simulink model "tb_CameraIO"  (R2022b)
settings: Solver=FixedStepDiscrete  StartTime=0  StopTime=0.0001  RelTol=1e-3
InitFcn:
  | init_CameraIO;
values from neighbouring files (symbols this model uses):
  AXI_CameraIO_Control = Simulink.Parameter    [init_CameraIO.m]
  model_time_step = 1/80e6    (= 1.25e-08)    [init_CameraIO.m]    (also in init_SYSTEM.m)
libraries: simulink x45, hdlsllib x13
Description:
  | Copyright (c) 2023, Alexei Evsenin, evsenin@gmail.com
settings Model: DataTypeOverride=Off  PacingRate=0.011000  Creator=mmwoperator  LastModifiedBy=evsenin
settings SolverCC: AlgebraicLoopSolver=TrustRegion
settings DataIOCC: SaveOutput=off  DSMLogging=off  SaveTime=off  ReturnWorkspaceOutputs=off
settings OptimizationCC: BlockReduction=off  ConditionallyExecuteInputs=off  DefaultParameterBehavior=Inlined  InheritOutputTypeSmallerThanSingle=on  DefaultUnderspecifiedDataType=single
settings DebuggingCC: AlgebraicLoopMsg=error  SingleTaskRateTransMsg=error  ParameterUnderflowMsg=error  ParameterPrecisionLossMsg=none  ParameterTunabilityLossMsg=error  FixptConstUnderflowMsg=warning  FixptConstOverflowMsg=warning  UnconnectedInputMsg=warning  UnconnectedOutputMsg=warning  UnconnectedLineMsg=warning  SFMachineParentedDataDiag=warning  UnderSpecifiedDimensionMsg=warning
settings HardwareCC: ProdBitPerPointer=32  ProdBitPerSizeT=32  ProdBitPerPtrDiffT=32  ProdLargestAtomicFloat=None  ProdIntDivRoundTo=Undefined  ProdEndianess=Unspecified  ProdWordSize=32  ProdHWDeviceType=ASIC/FPGA->ASIC/FPGA  TargetBitPerPointer=64  TargetBitPerSizeT=64  TargetBitPerPtrDiffT=64  TargetLongLongMode=on  TargetIntDivRoundTo=Zero  TargetEndianess=LittleEndian  TargetWordSize=64  TargetHWDeviceType=Custom Processor->MATLAB Host Computer  ProdEqTarget=off
settings ModelReferenceCC: EnableRefExpFcnMdlSchedulingChecks=on
settings RTWCC: DLArmComputeVersion=19.05

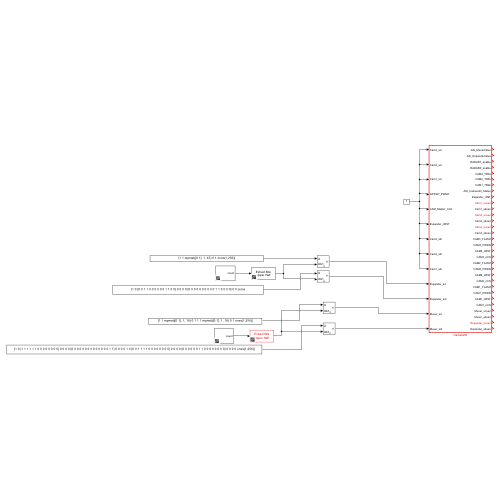
[thumbnail: Simulink's stored preview of the top-level diagram]
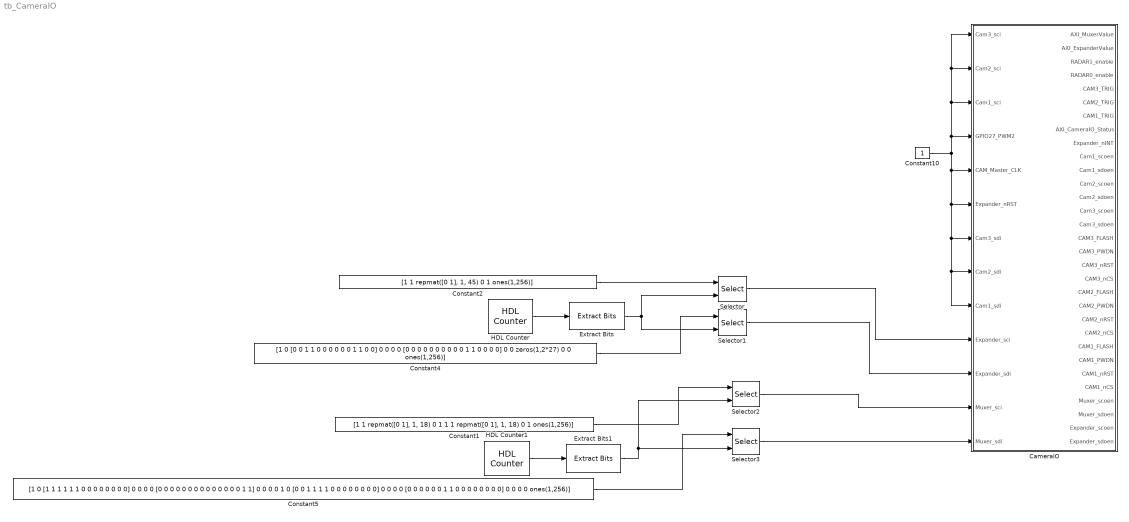
== system tb_CameraIO ==
  CameraIO : Subsystem  TreatAsAtomicUnit=on  SystemSampleTime=model_time_step
      settings: RTWSystemCode=Inline
  Constant1 : Constant  Value=[1 1 repmat([0 1], 1, 18) 0 1 1 1 repmat([0 1], 1, 18) 0 1 ones(1,256)]  OutDataTypeStr=boolean  SampleTime=model_time_step
  Constant10 : Constant  OutDataTypeStr=boolean  SampleTime=-1
  Constant2 : Constant  Value=[1 1 repmat([0 1], 1, 45) 0 1 ones(1,256)]  OutDataTypeStr=boolean  SampleTime=model_time_step
  Constant4 : Constant  Value="[1 0 [0 0 1 1 0 0 0 0 0 0 1 1 0 0] 0 0 0 0 [0 0 0 0 0 0 0 0 0 0 1 1 0 0 0 0] 0 0 zeros(1,2*27)  0 0 ones(1,256)]"  OutDataTypeStr=boolean  SampleTime=model_time_step
  Constant5 : Constant  Value=[1 0 [1 1 1 1 1 1 0 0 0 0 0 0 0 0] 0 0 0 0 [0 0 0 0 0 0 0 0 0 0 0 0 0 0 1 1] 0 0 0 0 1 0 [0 0 1 1 1 1 0 0 0 0 0 0 0 0] 0 0 0 0 [0 0 0 0 0 0 1 1 0 0 0 0 0 0 0 0] 0 0 0 0 ones(1,256)]  OutDataTypeStr=boolean  SampleTime=model_time_step
  Extract Bits : simulink/Logic and Bit Operations/Extract Bits  bitsToExtract=Upper half  numBits=8  bitIdxRange=[0 7]  outScalingMode=Treat bit field as an integer
  Extract Bits1 : simulink/Logic and Bit Operations/Extract Bits  bitsToExtract=Upper half  numBits=8  bitIdxRange=[0 7]  outScalingMode=Treat bit field as an integer
  HDL Counter : hdlsllib/Sources/HDL Counter  CountType=Free running  CountInit=0  CountStep=1  CountMax=25  CountFromType=Initial value  CountFrom=0  CountResetPort=off  CountLoadPort=off  CountEnbPort=off  CountDirPort=off  CountHitOutputPort=off  CountDataType=Unsigned  CountWordLen=16  CountFracLen=0  CountSampTime=model_time_step
  HDL Counter1 : hdlsllib/Sources/HDL Counter  CountType=Free running  CountInit=0  CountStep=1  CountMax=25  CountFromType=Initial value  CountFrom=0  CountResetPort=off  CountLoadPort=off  CountEnbPort=off  CountDirPort=off  CountHitOutputPort=off  CountDataType=Unsigned  CountWordLen=16  CountFracLen=0  CountSampTime=model_time_step
  Selector{,1..3} (4 alike) : Selector  IndexMode=Zero-based  IndexOptions=Index vector (port)  Indices=[1 3]  OutputSizes=1
  wires:
  Constant2/1 -> Selector/1
  Selector/1 -> CameraIO/4(Expander_sci)
  Selector1/1 -> CameraIO/3(Expander_sdi)
  Extract Bits/1 -> Selector1/2, Selector/2
  Constant4/1 -> Selector1/1
  HDL Counter/1 -> Extract Bits/1
  Extract Bits1/1 -> Selector3/2, Selector2/2
  Selector3/1 -> CameraIO/1(Muxer_sdi)
  Selector2/1 -> CameraIO/2(Muxer_sci)
  Constant1/1 -> Selector2/1
  Constant5/1 -> Selector3/1
  HDL Counter1/1 -> Extract Bits1/1
  Constant10/1 -> CameraIO/5(Cam1_sdi), CameraIO/6(Cam2_sdi), CameraIO/7(Cam3_sdi), CameraIO/8(Expander_nRST), CameraIO/9(CAM_Master_CLK), CameraIO/13(Cam3_sci), CameraIO/12(Cam2_sci), CameraIO/11(Cam1_sci), CameraIO/10(GPIO27_PWM2)

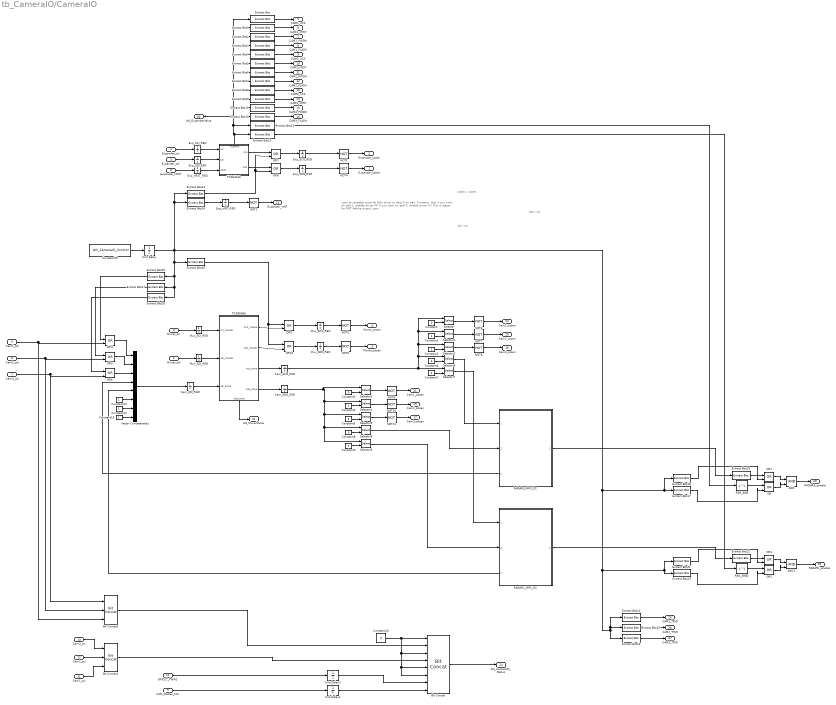
== system tb_CameraIO/CameraIO ==
  note: sdoen /
      | scoen
  note: _oen pin enables external bidir driver to pass 0 on pad.
      | It means, that
      | if you want on pad 1, disable driver (0)
      | if you want on pad 0, enable driver (1)
      | This is reason for NOT before output _oen
  note: sdi /
      | sci
  note: sda /
      | scl
  Muxer_sdi : Inport
  Muxer_sci : Inport  Port=2
  Expander_sdi : Inport  Port=3
  Expander_sci : Inport  Port=4
  Cam1_sdi : Inport  Port=5
  Cam2_sdi : Inport  Port=6
  Cam3_sdi : Inport  Port=7
  Expander_nRST : Inport  Port=8
  CAM_Master_CLK : Inport  Port=9
  GPIO27_PWM2 : Inport  Port=10
  Cam1_sci : Inport  Port=11
  Cam2_sci : Inport  Port=12
  Cam3_sci : Inport  Port=13
  AND : Logic  IconShape=distinctive  AllPortsSameDT=off  OutDataTypeStr=boolean
  AND1 : Logic  IconShape=distinctive  AllPortsSameDT=off  OutDataTypeStr=boolean
  Bit Concat : hdlsllib/Logic and Bit Operations/Bit Concat  numInputs=8
  Bit Concat1 : hdlsllib/Logic and Bit Operations/Bit Concat  numInputs=3
  Bit Concat2 : hdlsllib/Logic and Bit Operations/Bit Concat  numInputs=3
  Cam_SCO_REG : UnitDelay  SampleTime=-1  HasFrameUpgradeWarning=on
  Cam_SDI_REG : UnitDelay  SampleTime=-1  HasFrameUpgradeWarning=on
  Cam_SDO_REG : UnitDelay  SampleTime=-1  HasFrameUpgradeWarning=on
  Constant : Constant  Value=0  OutDataTypeStr=uint8  SampleTime=-1
  Constant1 : Constant  OutDataTypeStr=uint8  SampleTime=-1
  Constant10 : Constant  Value=0  OutDataTypeStr=boolean  SampleTime=-1
  Constant13 : Constant  OutDataTypeStr=boolean  SampleTime=-1
  Constant14 : Constant  OutDataTypeStr=boolean  SampleTime=-1
  Constant15 : Constant  OutDataTypeStr=boolean  SampleTime=-1
  Constant19 : Constant  Value=AXI_CameraIO_Control  SampleTime=-1
  Constant2 : Constant  Value=2  OutDataTypeStr=uint8  SampleTime=-1
  Constant3 : Constant  Value=0  OutDataTypeStr=uint8  SampleTime=-1
  Constant4 : Constant  OutDataTypeStr=uint8  SampleTime=-1
  Constant5 : Constant  Value=2  OutDataTypeStr=uint8  SampleTime=-1
  Constant6 : Constant  Value=3  OutDataTypeStr=uint8  SampleTime=-1
  Constant7 : Constant  Value=4  OutDataTypeStr=uint8  SampleTime=-1
  Constant8 : Constant  Value=3  OutDataTypeStr=uint8  SampleTime=-1
  Constant9 : Constant  Value=4  OutDataTypeStr=uint8  SampleTime=-1
  Exp_SCI_REG : UnitDelay  SampleTime=-1  HasFrameUpgradeWarning=on
  Exp_SCO_REG : UnitDelay  SampleTime=-1  HasFrameUpgradeWarning=on
  Exp_SDI_REG : UnitDelay  SampleTime=-1  HasFrameUpgradeWarning=on
  Exp_SDO_REG : UnitDelay  SampleTime=-1  HasFrameUpgradeWarning=on
  Exp_nINT_REG : UnitDelay  SampleTime=-1  HasFrameUpgradeWarning=on
  Exp_nRST_REG : UnitDelay  SampleTime=-1  HasFrameUpgradeWarning=on
  Extract Bits : simulink/Logic and Bit Operations/Extract Bits  bitsToExtract=Range of bits  numBits=8  bitIdxRange=0  outScalingMode=Treat bit field as an integer
  Extract Bits1 : simulink/Logic and Bit Operations/Extract Bits  bitsToExtract=Range of bits  numBits=8  bitIdxRange=1  outScalingMode=Treat bit field as an integer
  Extract Bits10 : simulink/Logic and Bit Operations/Extract Bits  bitsToExtract=Range of bits  numBits=8  bitIdxRange=11  outScalingMode=Treat bit field as an integer
  Extract Bits11 : simulink/Logic and Bit Operations/Extract Bits  bitsToExtract=Range of bits  numBits=8  bitIdxRange=12  outScalingMode=Treat bit field as an integer
  Extract Bits12 : simulink/Logic and Bit Operations/Extract Bits  bitsToExtract=Range of bits  numBits=8  bitIdxRange=13  outScalingMode=Treat bit field as an integer
  Extract Bits13 : simulink/Logic and Bit Operations/Extract Bits  bitsToExtract=Range of bits  numBits=8  bitIdxRange=14  outScalingMode=Treat bit field as an integer
  Extract Bits14 : simulink/Logic and Bit Operations/Extract Bits  bitsToExtract=Range of bits  numBits=8  bitIdxRange=1  outScalingMode=Treat bit field as an integer
  Extract Bits15 : simulink/Logic and Bit Operations/Extract Bits  bitsToExtract=Range of bits  numBits=8  bitIdxRange=2  outScalingMode=Treat bit field as an integer
  Extract Bits16 : simulink/Logic and Bit Operations/Extract Bits  bitsToExtract=Range of bits  numBits=8  bitIdxRange=3  outScalingMode=Treat bit field as an integer
  Extract Bits17 : simulink/Logic and Bit Operations/Extract Bits  bitsToExtract=Range of bits  numBits=8  bitIdxRange=10  outScalingMode=Treat bit field as an integer
  Extract Bits18 : simulink/Logic and Bit Operations/Extract Bits  bitsToExtract=Range of bits  numBits=8  bitIdxRange=11  outScalingMode=Treat bit field as an integer
  Extract Bits19 : simulink/Logic and Bit Operations/Extract Bits  bitsToExtract=Range of bits  numBits=8  bitIdxRange=0  outScalingMode=Treat bit field as an integer
  Extract Bits2 : simulink/Logic and Bit Operations/Extract Bits  bitsToExtract=Range of bits  numBits=8  bitIdxRange=2  outScalingMode=Treat bit field as an integer
  Extract Bits20 : simulink/Logic and Bit Operations/Extract Bits  bitsToExtract=Range of bits  numBits=8  bitIdxRange=8  outScalingMode=Treat bit field as an integer
  Extract Bits21 : simulink/Logic and Bit Operations/Extract Bits  bitsToExtract=Range of bits  numBits=8  bitIdxRange=9  outScalingMode=Treat bit field as an integer
  Extract Bits22 : simulink/Logic and Bit Operations/Extract Bits  bitsToExtract=Range of bits  numBits=8  bitIdxRange=0  outScalingMode=Treat bit field as an integer
  Extract Bits23 : simulink/Logic and Bit Operations/Extract Bits  bitsToExtract=Range of bits  numBits=8  bitIdxRange=16  outScalingMode=Treat bit field as an integer
  Extract Bits24 : simulink/Logic and Bit Operations/Extract Bits  bitsToExtract=Range of bits  numBits=8  bitIdxRange=17  outScalingMode=Treat bit field as an integer
  Extract Bits25 : simulink/Logic and Bit Operations/Extract Bits  bitsToExtract=Range of bits  numBits=8  bitIdxRange=24  outScalingMode=Treat bit field as an integer
  Extract Bits26 : simulink/Logic and Bit Operations/Extract Bits  bitsToExtract=Range of bits  numBits=8  bitIdxRange=20  outScalingMode=Treat bit field as an integer
  Extract Bits27 : simulink/Logic and Bit Operations/Extract Bits  bitsToExtract=Range of bits  numBits=8  bitIdxRange=25  outScalingMode=Treat bit field as an integer
  Extract Bits28 : simulink/Logic and Bit Operations/Extract Bits  bitsToExtract=Range of bits  numBits=8  bitIdxRange=26  outScalingMode=Treat bit field as an integer
  Extract Bits3 : simulink/Logic and Bit Operations/Extract Bits  bitsToExtract=Range of bits  numBits=8  bitIdxRange=3  outScalingMode=Treat bit field as an integer
  Extract Bits4 : simulink/Logic and Bit Operations/Extract Bits  bitsToExtract=Range of bits  numBits=8  bitIdxRange=5  outScalingMode=Treat bit field as an integer
  Extract Bits5 : simulink/Logic and Bit Operations/Extract Bits  bitsToExtract=Range of bits  numBits=8  bitIdxRange=6  outScalingMode=Treat bit field as an integer
  Extract Bits6 : simulink/Logic and Bit Operations/Extract Bits  bitsToExtract=Range of bits  numBits=8  bitIdxRange=7  outScalingMode=Treat bit field as an integer
  Extract Bits7 : simulink/Logic and Bit Operations/Extract Bits  bitsToExtract=Range of bits  numBits=8  bitIdxRange=8  outScalingMode=Treat bit field as an integer
  Extract Bits8 : simulink/Logic and Bit Operations/Extract Bits  bitsToExtract=Range of bits  numBits=8  bitIdxRange=9  outScalingMode=Treat bit field as an integer
  Extract Bits9 : simulink/Logic and Bit Operations/Extract Bits  bitsToExtract=Range of bits  numBits=8  bitIdxRange=10  outScalingMode=Treat bit field as an integer
  Mux_SCI_REG : UnitDelay  SampleTime=-1  HasFrameUpgradeWarning=on
  Mux_SCO_REG : UnitDelay  SampleTime=-1  HasFrameUpgradeWarning=on
  Mux_SDI_REG : UnitDelay  SampleTime=-1  HasFrameUpgradeWarning=on
  Mux_SDO_REG : UnitDelay  SampleTime=-1  HasFrameUpgradeWarning=on
  NOT{1..11} (11 alike) : Logic  Operator=NOT  IconShape=distinctive  AllPortsSameDT=off  OutDataTypeStr=boolean
  OR{,1..10} (11 alike) : Logic  Operator=OR  IconShape=distinctive  AllPortsSameDT=off  OutDataTypeStr=boolean
  RADAR0_MIPI_I2C : Subsystem  ReferencedSubsystem=RADAR_MIPI_I2C
      settings: PortSchema="{\"entries\":[{\"content\":{\"sides\":[{\"content\":{\"connectorIds\":[\"In1\",\"In2\",\"Out2\"]},\"type\":\"ConnectorPlacement.EquallySpacedRectSide\",\"uuid\":\"b2debd9d-8b2d-4c2a-b7ea-d85f4bcb52c2\"},{\"content\":{\"connectorIds\":[\"Out1\"],\"side\":\"RIGHT\"},\"type\":\"ConnectorPlacement.EquallySpacedRectSide\",\"uuid\":\"751dea3d-0503-49a0-b2b7-e7f0bb60b899\"},{\"content\":{\"connectorIds\":[],\"side\":\"TOP\"},\"type\":\"ConnectorPlacement.EquallySpacedRectSide\",\"uuid\":\"f461e2eb-1348-46d1-881b-f4de32057164\"}]},\"type\":\"ConnectorPlacement.EquallySpacedConnector\",\"uuid\":\"9a0ee4b4-c8e7-4064-9f6e-581825dbb5da\"}],\"packageUris\":[\"http://schema.mathworks.com/mf0/Connector/R2020b\"],\"version\":\"1.0\"}"
  RADAR1_MIPI_I2C : Subsystem  ReferencedSubsystem=RADAR_MIPI_I2C
      settings: PortSchema="{\"entries\":[{\"content\":{\"sides\":[{\"content\":{\"connectorIds\":[\"In1\",\"In2\",\"Out2\"]},\"type\":\"ConnectorPlacement.EquallySpacedRectSide\",\"uuid\":\"b2debd9d-8b2d-4c2a-b7ea-d85f4bcb52c2\"},{\"content\":{\"connectorIds\":[\"Out1\"],\"side\":\"RIGHT\"},\"type\":\"ConnectorPlacement.EquallySpacedRectSide\",\"uuid\":\"751dea3d-0503-49a0-b2b7-e7f0bb60b899\"},{\"content\":{\"connectorIds\":[],\"side\":\"TOP\"},\"type\":\"ConnectorPlacement.EquallySpacedRectSide\",\"uuid\":\"f461e2eb-1348-46d1-881b-f4de32057164\"}]},\"type\":\"ConnectorPlacement.EquallySpacedConnector\",\"uuid\":\"9a0ee4b4-c8e7-4064-9f6e-581825dbb5da\"}],\"packageUris\":[\"http://schema.mathworks.com/mf0/Connector/R2020b\"],\"version\":\"1.0\"}"
  REG_ENB : Delay  DelayLength=1
  REG_ENB1 : Delay  DelayLength=1
  Selector{,1..9} (10 alike) : Selector  IndexMode=Zero-based  IndexOptions=Index vector (port)  Indices=0  OutputSizes=1
  TCA6424A : Subsystem
      settings: PortSchema="{\"entries\":[{\"content\":{\"sides\":[{\"content\":{\"connectorIds\":[\"In1\",\"In2\",\"In3\"]},\"type\":\"ConnectorPlacement.EquallySpacedRectSide\",\"uuid\":\"1d77250f-43b6-4386-b675-1e83793e08db\"},{\"content\":{\"connectorIds\":[\"Out1\",\"Out2\"],\"side\":\"RIGHT\"},\"type\":\"ConnectorPlacement.EquallySpacedRectSide\",\"uuid\":\"1b640580-4115-4d83-96ca-02609d981243\"},{\"content\":{\"connectorIds\":[\"Out3\"],\"side\":\"TOP\"},\"type\":\"ConnectorPlacement.EquallySpacedRectSide\",\"uuid\":\"6f49e433-be00-44ee-960e-7edaa7f3e149\"},{\"content\":{\"connectorIds\":[],\"side\":\"BOTTOM\"},\"type\":\"ConnectorPlacement.EquallySpacedRectSide\",\"uuid\":\"6a3152cf-8f3f-4f35-b098-7ea6aba78185\"}]},\"type\":\"ConnectorPlacement.EquallySpacedConnector\",\"uuid\":\"cd4e3591-6f3d-41af-8f32-177195735550\"}],\"packageUris\":[\"http://schema.mathworks.com/mf0/Connector/R2020b\"],\"version\":\"1.0\"}"
  TCA9548A : Subsystem
      settings: PortSchema="{\"entries\":[{\"content\":{\"sides\":[{\"content\":{\"connectorIds\":[\"In1\",\"In2\",\"In3\"]},\"type\":\"ConnectorPlacement.EquallySpacedRectSide\",\"uuid\":\"30138089-1687-4fa9-aa54-8d9fb6e280a7\"},{\"content\":{\"connectorIds\":[\"Out1\",\"Out2\",\"Out3\",\"Out4\"],\"side\":\"RIGHT\"},\"type\":\"ConnectorPlacement.EquallySpacedRectSide\",\"uuid\":\"5e979874-09c9-45f9-a69c-4ffe93cd782d\"},{\"content\":{\"connectorIds\":[],\"side\":\"TOP\"},\"type\":\"ConnectorPlacement.EquallySpacedRectSide\",\"uuid\":\"c2d29317-3627-4549-aad4-654ad2aeb24a\"},{\"content\":{\"connectorIds\":[\"Out5\"],\"side\":\"BOTTOM\"},\"type\":\"ConnectorPlacement.EquallySpacedRectSide\",\"uuid\":\"d73dba4d-9b9b-4bcf-9d79-4dc188f6521f\"}]},\"type\":\"ConnectorPlacement.EquallySpacedConnector\",\"uuid\":\"ba77235e-1c79-4f82-b9b9-043309a3d168\"}],\"packageUris\":[\"http://schema.mathworks.com/mf0/Connector/R2020b\"],\"version\":\"1.0\"}"
  Unit Delay : UnitDelay  SampleTime=-1  HasFrameUpgradeWarning=on
  Unit Delay1 : UnitDelay  SampleTime=-1  HasFrameUpgradeWarning=on
  Unit Delay2 : UnitDelay  SampleTime=-1  HasFrameUpgradeWarning=on
  Vector Concatenate1 : Concatenate  NumInputs=8
  Expander_sdoen : Outport
  Expander_scoen : Outport  Port=2
  Muxer_sdoen : Outport  Port=3
  Muxer_scoen : Outport  Port=4
  CAM1_nCS : Outport  Port=5
  CAM1_nRST : Outport  Port=6
  CAM1_PWDN : Outport  Port=7
  CAM1_FLASH : Outport  Port=8
  CAM2_nCS : Outport  Port=9
  CAM2_nRST : Outport  Port=10
  CAM2_PWDN : Outport  Port=11
  CAM2_FLASH : Outport  Port=12
  CAM3_nCS : Outport  Port=13
  CAM3_nRST : Outport  Port=14
  CAM3_PWDN : Outport  Port=15
  CAM3_FLASH : Outport  Port=16
  Cam3_sdoen : Outport  Port=17
  Cam3_scoen : Outport  Port=18
  Cam2_sdoen : Outport  Port=19
  Cam2_scoen : Outport  Port=20
  Cam1_sdoen : Outport  Port=21
  Cam1_scoen : Outport  Port=22
  Expander_nINT : Outport  Port=23
  AXI_CameraIO_Status : Outport  Port=24
  CAM1_TRIG : Outport  Port=25
  CAM2_TRIG : Outport  Port=26
  CAM3_TRIG : Outport  Port=27
  RADAR0_enable : Outport  Port=28
  RADAR1_enable : Outport  Port=29
  AXI_ExpanderValue : Outport  Port=30
  AXI_MuxerValue : Outport  Port=31
  wires:
  Expander_sci/1 -> Exp_SCI_REG/1
  Expander_sdi/1 -> Exp_SDI_REG/1
  Muxer_sci/1 -> Mux_SCI_REG/1
  Muxer_sdi/1 -> Mux_SDI_REG/1
  Extract Bits/1 -> CAM1_nCS/1
  Extract Bits1/1 -> CAM1_nRST/1
  Extract Bits2/1 -> CAM1_PWDN/1
  Extract Bits3/1 -> CAM1_FLASH/1
  Extract Bits6/1 -> CAM2_PWDN/1
  Extract Bits7/1 -> CAM2_FLASH/1
  Extract Bits5/1 -> CAM2_nRST/1
  Extract Bits4/1 -> CAM2_nCS/1
  Extract Bits9/1 -> CAM3_nRST/1
  Extract Bits10/1 -> CAM3_PWDN/1
  Extract Bits8/1 -> CAM3_nCS/1
  Extract Bits11/1 -> CAM3_FLASH/1
  Extract Bits13/1 -> REG_ENB1/1
  Extract Bits12/1 -> REG_ENB/1
  TCA6424A/3(OutPort) -> AXI_ExpanderValue/1, Extract Bits/1, Extract Bits1/1, Extract Bits2/1, Extract Bits3/1, Extract Bits4/1, Extract Bits5/1, Extract Bits6/1, Extract Bits7/1, Extract Bits8/1, Extract Bits9/1, Extract Bits10/1, Extract Bits11/1, Extract Bits12/1, Extract Bits13/1
  Selector/1 -> NOT6/1
  Constant/1 -> Selector/2
  Constant1/1 -> Selector1/2
  Selector1/1 -> NOT7/1
  Selector2/1 -> NOT8/1
  Constant2/1 -> Selector2/2
  Constant5/1 -> Selector5/2
  Constant3/1 -> Selector3/2
  Selector3/1 -> NOT9/1
  Constant4/1 -> Selector4/2
  Selector5/1 -> NOT11/1
  Selector4/1 -> NOT10/1
  TCA9548A/3(sco_slave) -> Cam_SCO_REG/1
  Constant7/1 -> Selector7/2
  Constant6/1 -> Selector6/2
  TCA9548A/4(sdo_slave) -> Cam_SDO_REG/1
  Constant8/1 -> Selector8/2
  Constant9/1 -> Selector9/2
  Constant13/1 -> Vector Concatenate1/6
  Cam3_sdi/1 -> Bit Concat2/1, OR6/2
  Constant15/1 -> Vector Concatenate1/8
  Constant14/1 -> Vector Concatenate1/7
  Cam2_sdi/1 -> Bit Concat2/2, OR5/2
  Vector Concatenate1/1 -> Cam_SDI_REG/1
  Selector6/1 -> RADAR0_MIPI_I2C/1
  Selector8/1 -> RADAR0_MIPI_I2C/2
  RADAR0_MIPI_I2C/1 -> Extract Bits19/1
  RADAR0_MIPI_I2C/2 -> Vector Concatenate1/4
  RADAR1_MIPI_I2C/1 -> Extract Bits22/1
  Selector9/1 -> RADAR1_MIPI_I2C/2
  Selector7/1 -> RADAR1_MIPI_I2C/1
  RADAR1_MIPI_I2C/2 -> Vector Concatenate1/5
  Expander_nRST/1 -> Exp_nRST_REG/1
  Extract Bits24/1 -> Exp_nINT_REG/1
  Constant19/1 -> Unit Delay/1
  Extract Bits14/1 -> CAM1_TRIG/1
  Extract Bits15/1 -> CAM2_TRIG/1
  Extract Bits16/1 -> CAM3_TRIG/1
  CAM_Master_CLK/1 -> Unit Delay1/1
  GPIO27_PWM2/1 -> Unit Delay2/1
  Bit Concat/1 -> AXI_CameraIO_Status/1
  OR/1 -> AND/2
  Extract Bits17/1 -> OR/2
  REG_ENB/1 -> OR/1
  Extract Bits19/1 -> OR1/1
  Extract Bits18/1 -> OR1/2
  OR1/1 -> AND/1
  Extract Bits20/1 -> OR2/2
  OR2/1 -> AND1/2
  OR3/1 -> AND1/1
  Extract Bits21/1 -> OR3/2
  REG_ENB1/1 -> OR2/1
  Extract Bits22/1 -> OR3/1
  Unit Delay/1 -> Extract Bits28/1, Extract Bits27/1, Extract Bits25/1, Extract Bits26/1, Extract Bits24/1, Extract Bits23/1, Extract Bits16/1, Extract Bits14/1, Extract Bits15/1, Extract Bits21/1, Extract Bits20/1, Extract Bits18/1, Extract Bits17/1
  AND/1 -> RADAR0_enable/1
  AND1/1 -> RADAR1_enable/1
  Exp_SCI_REG/1 -> TCA6424A/1(sci)
  Exp_SDI_REG/1 -> TCA6424A/2(sdi)
  Exp_SCO_REG/1 -> NOT1/1
  Exp_SDO_REG/1 -> NOT4/1
  Exp_nRST_REG/1 -> TCA6424A/3(nRST)
  Mux_SCI_REG/1 -> TCA9548A/1(sci_master)
  Mux_SDI_REG/1 -> TCA9548A/2(sdi_master)
  Mux_SCO_REG/1 -> NOT3/1
  Mux_SDO_REG/1 -> NOT5/1
  Cam_SDI_REG/1 -> TCA9548A/3(sdi_slave)
  Cam_SCO_REG/1 -> Selector1/1, Selector/1, Selector2/1, Selector6/1, Selector7/1
  Cam_SDO_REG/1 -> Selector3/1, Selector8/1, Selector9/1, Selector5/1, Selector4/1
  Extract Bits23/1 -> OR8/2, OR7/2
  TCA6424A/1(sco) -> OR7/1
  OR7/1 -> Exp_SCO_REG/1
  TCA6424A/2(sdo) -> OR8/1
  OR8/1 -> Exp_SDO_REG/1
  Exp_nINT_REG/1 -> NOT2/1
  Extract Bits26/1 -> OR10/1, OR9/1
  OR9/1 -> Mux_SCO_REG/1
  TCA9548A/1(sco_master) -> OR9/2
  OR10/1 -> Mux_SDO_REG/1
  TCA9548A/2(sdo_master) -> OR10/2
  Extract Bits25/1 -> OR4/1
  Cam1_sdi/1 -> Bit Concat2/3, OR4/2
  OR4/1 -> Vector Concatenate1/1
  OR5/1 -> Vector Concatenate1/2
  Extract Bits27/1 -> OR5/1
  OR6/1 -> Vector Concatenate1/3
  Extract Bits28/1 -> OR6/1
  NOT1/1 -> Expander_scoen/1
  NOT4/1 -> Expander_sdoen/1
  NOT2/1 -> Expander_nINT/1
  NOT3/1 -> Muxer_scoen/1
  NOT5/1 -> Muxer_sdoen/1
  NOT6/1 -> Cam1_scoen/1
  NOT7/1 -> Cam2_scoen/1
  NOT8/1 -> Cam3_scoen/1
  NOT9/1 -> Cam1_sdoen/1
  NOT10/1 -> Cam2_sdoen/1
  NOT11/1 -> Cam3_sdoen/1
  TCA9548A/5(last_byte) -> AXI_MuxerValue/1
  Cam1_sci/1 -> Bit Concat1/3
  Cam2_sci/1 -> Bit Concat1/2
  Cam3_sci/1 -> Bit Concat1/1
  Bit Concat2/1 -> Bit Concat/2
  Unit Delay1/1 -> Bit Concat/8
  Unit Delay2/1 -> Bit Concat/7
  Bit Concat1/1 -> Bit Concat/4
  Constant10/1 -> Bit Concat/1, Bit Concat/3, Bit Concat/5, Bit Concat/6

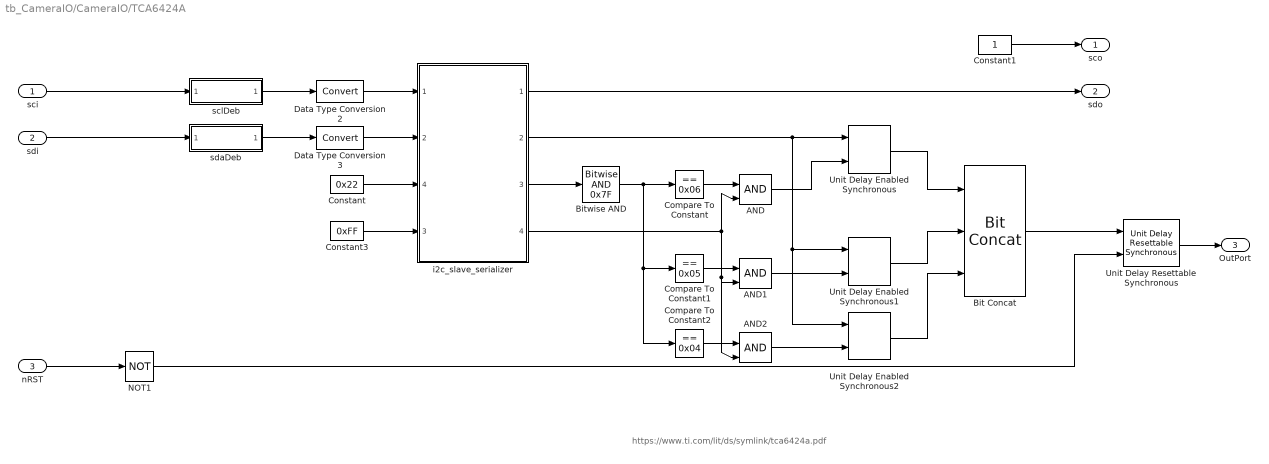
== system tb_CameraIO/CameraIO/TCA6424A ==
  note: https://www.ti.com/lit/ds/symlink/tca6424a.pdf
  sci : Inport
  sdi : Inport  Port=2
  nRST : Inport  Port=3
  AND : Logic  IconShape=distinctive  AllPortsSameDT=off  OutDataTypeStr=boolean
  AND1 : Logic  IconShape=distinctive  AllPortsSameDT=off  OutDataTypeStr=boolean
  AND2 : Logic  IconShape=distinctive  AllPortsSameDT=off  OutDataTypeStr=boolean
  Bit Concat : hdlsllib/Logic and Bit Operations/Bit Concat  numInputs=3
  Bitwise AND : simulink/Logic and Bit Operations/Bitwise Operator  logicop=AND  UseBitMask=on  BitMask=0x7F  BitMaskRealWorld=Stored Integer
  Compare To Constant : simulink/Logic and Bit Operations/Compare To Constant  relop===  const=0x06  OutDataTypeStr=boolean
  Compare To Constant1 : simulink/Logic and Bit Operations/Compare To Constant  relop===  const=0x05  OutDataTypeStr=boolean
  Compare To Constant2 : simulink/Logic and Bit Operations/Compare To Constant  relop===  const=0x04  OutDataTypeStr=boolean
  Constant : Constant  Value=0x22  OutDataTypeStr=fixdt(0,7,0)  SampleTime=-1
  Constant1 : Constant  OutDataTypeStr=boolean  SampleTime=-1
  Constant3 : Constant  Value=0xFF  OutDataTypeStr=uint8  SampleTime=-1
  Data Type Conversion2 : DataTypeConversion  SaturateOnIntegerOverflow=off  RndMeth=Floor
  Data Type Conversion3 : DataTypeConversion  SaturateOnIntegerOverflow=off  RndMeth=Floor
  NOT1 : Logic  Operator=NOT  IconShape=distinctive  AllPortsSameDT=off  OutDataTypeStr=boolean
  Unit Delay Enabled Synchronous : hdlsllib/Discrete/Unit Delay Enabled Synchronous  InitialCondition=0xFF  SampleTime=-1
  Unit Delay Enabled Synchronous1 : hdlsllib/Discrete/Unit Delay Enabled Synchronous  InitialCondition=0xFF  SampleTime=-1
  Unit Delay Enabled Synchronous2 : hdlsllib/Discrete/Unit Delay Enabled Synchronous  InitialCondition=0xFF  SampleTime=-1
  Unit Delay Resettable Synchronous : hdlsllib/Discrete/Unit Delay Resettable Synchronous  InitialCondition=1  SampleTime=-1
  i2c_slave_serializer : Subsystem  ReferencedSubsystem=i2c_slave_serializer
      settings: PortSchema="{\"entries\":[{\"content\":{\"sides\":[{\"content\":{\"connectorIds\":[\"In1\",\"In2\",\"In4\",\"In3\"]},\"type\":\"ConnectorPlacement.EquallySpacedRectSide\",\"uuid\":\"5cabedeb-c807-4889-8ba0-5ab9031a84ba\"},{\"content\":{\"connectorIds\":[\"Out1\",\"Out2\",\"Out3\",\"Out4\"],\"side\":\"RIGHT\"},\"type\":\"ConnectorPlacement.EquallySpacedRectSide\",\"uuid\":\"ca7acdc8-82b2-4681-aa13-89f67544921e\"},{\"content\":{\"connectorIds\":[],\"side\":\"TOP\"},\"type\":\"ConnectorPlacement.EquallySpacedRectSide\",\"uuid\":\"8b24d124-fa07-455d-a189-f258fbea822f\"}]},\"type\":\"ConnectorPlacement.EquallySpacedConnector\",\"uuid\":\"6802f4c9-cf5e-4fdc-ad1f-26d27f7bb24e\"}],\"packageUris\":[\"http://schema.mathworks.com/mf0/Connector/R2020b\"],\"version\":\"1.0\"}"
  sclDeb : Subsystem  ReferencedSubsystem=debounce
  sdaDeb : Subsystem  ReferencedSubsystem=debounce
  sco : Outport
  sdo : Outport  Port=2
  OutPort : Outport  Port=3
  wires:
  Constant3/1 -> i2c_slave_serializer/3
  sclDeb/1 -> Data Type Conversion2/1
  Data Type Conversion3/1 -> i2c_slave_serializer/2
  Constant/1 -> i2c_slave_serializer/4
  sdaDeb/1 -> Data Type Conversion3/1
  Data Type Conversion2/1 -> i2c_slave_serializer/1
  i2c_slave_serializer/3 -> Bitwise AND/1
  Compare To Constant/1 -> AND/1
  AND/1 -> Unit Delay Enabled Synchronous/2
  AND1/1 -> Unit Delay Enabled Synchronous1/2
  Compare To Constant1/1 -> AND1/1
  i2c_slave_serializer/4 -> AND2/2, AND1/2, AND/2
  Bitwise AND/1 -> Compare To Constant2/1, Compare To Constant1/1, Compare To Constant/1
  i2c_slave_serializer/2 -> Unit Delay Enabled Synchronous2/1, Unit Delay Enabled Synchronous1/1, Unit Delay Enabled Synchronous/1
  Compare To Constant2/1 -> AND2/1
  AND2/1 -> Unit Delay Enabled Synchronous2/2
  Unit Delay Enabled Synchronous2/1 -> Bit Concat/3
  Unit Delay Enabled Synchronous1/1 -> Bit Concat/2
  Unit Delay Enabled Synchronous/1 -> Bit Concat/1
  Bit Concat/1 -> Unit Delay Resettable Synchronous/1
  Constant1/1 -> sco/1
  i2c_slave_serializer/1 -> sdo/1
  Unit Delay Resettable Synchronous/1 -> OutPort/1
  sci/1 -> sclDeb/1
  sdi/1 -> sdaDeb/1
  nRST/1 -> NOT1/1
  NOT1/1 -> Unit Delay Resettable Synchronous/2

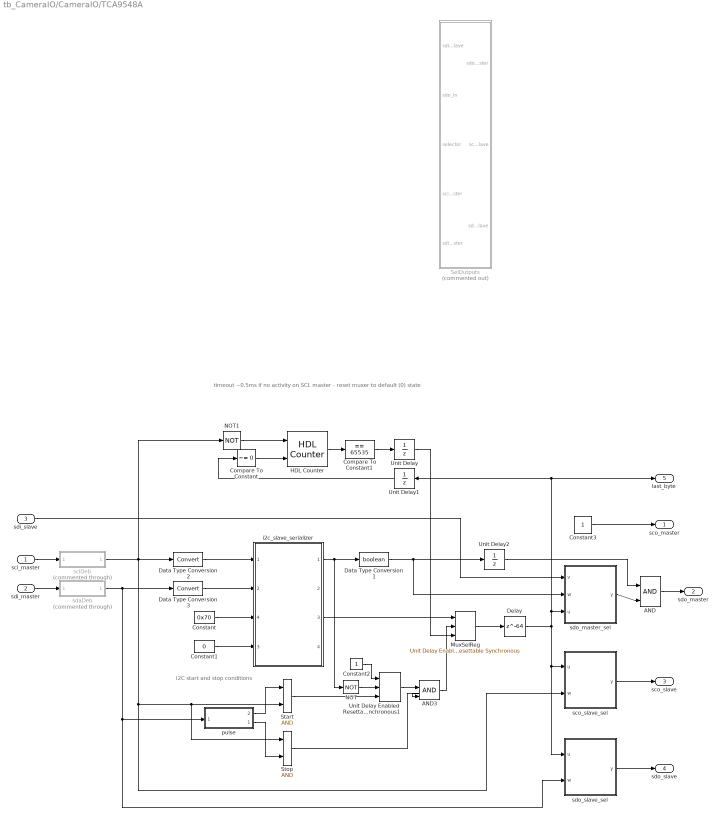
== system tb_CameraIO/CameraIO/TCA9548A ==
  note: timeout ~0.5ms if no activity on SCL master -
      | reset muxer to default (0) state
  note: I2C start and stop conditions
  sci_master : Inport
  sdi_master : Inport  Port=2
  sdi_slave : Inport  Port=3
  AND : Logic  IconShape=distinctive  AllPortsSameDT=off  OutDataTypeStr=boolean
  AND3 : Logic  IconShape=distinctive  AllPortsSameDT=off  OutDataTypeStr=boolean
  Compare To Constant : simulink/Logic and Bit Operations/Compare To Constant  relop=~=  const=0  OutDataTypeStr=boolean
  Compare To Constant1 : simulink/Logic and Bit Operations/Compare To Constant  relop===  const=65535  OutDataTypeStr=boolean
  Constant : Constant  Value=0x70  OutDataTypeStr=fixdt(0,7,0)  SampleTime=-1
  Constant1 : Constant  Value=0  OutDataTypeStr=uint8  SampleTime=-1
  Constant2 : Constant  OutDataTypeStr=boolean  SampleTime=-1
  Constant3 : Constant  OutDataTypeStr=boolean  SampleTime=-1
  Data Type Conversion1 : DataTypeConversion  OutDataTypeStr=boolean  SaturateOnIntegerOverflow=off  RndMeth=Floor
  Data Type Conversion2 : DataTypeConversion  SaturateOnIntegerOverflow=off  RndMeth=Floor
  Data Type Conversion3 : DataTypeConversion  SaturateOnIntegerOverflow=off  RndMeth=Floor
  Delay : Delay  DelayLength=64
  HDL Counter : hdlsllib/Sources/HDL Counter  CountType=Free running  CountInit=0  CountStep=1  CountMax=25  CountFromType=Initial value  CountFrom=0  CountResetPort=on  CountLoadPort=off  CountEnbPort=on  CountDirPort=off  CountHitOutputPort=off  CountDataType=Unsigned  CountWordLen=16  CountFracLen=0  CountSampTime=1
  MuxSelReg : hdlsllib/Discrete/Unit Delay Enabled Resettable Synchronous  InitialCondition=0  SampleTime=-1
  NOT : Logic  Operator=NOT  IconShape=distinctive  AllPortsSameDT=off  OutDataTypeStr=boolean
  NOT1 : Logic  Operator=NOT  IconShape=distinctive  AllPortsSameDT=off  OutDataTypeStr=boolean
  SelOutputs : Subsystem  Commented=on
  Start : Logic  IconShape=distinctive  AllPortsSameDT=off  OutDataTypeStr=boolean
  Stop : Logic  IconShape=distinctive  AllPortsSameDT=off  OutDataTypeStr=boolean
  Unit Delay : UnitDelay  SampleTime=-1  HasFrameUpgradeWarning=on
  Unit Delay Enabled Resettable Synchronous1 : hdlsllib/Discrete/Unit Delay Enabled Resettable Synchronous  InitialCondition=0  SampleTime=-1
  Unit Delay1 : UnitDelay  SampleTime=-1  HasFrameUpgradeWarning=on
  Unit Delay2 : UnitDelay  SampleTime=-1  HasFrameUpgradeWarning=on
  i2c_slave_serializer : Subsystem  ReferencedSubsystem=i2c_slave_serializer
      settings: PortSchema="{\"entries\":[{\"content\":{\"sides\":[{\"content\":{\"connectorIds\":[\"In1\",\"In2\",\"In4\",\"In3\"]},\"type\":\"ConnectorPlacement.EquallySpacedRectSide\",\"uuid\":\"5cabedeb-c807-4889-8ba0-5ab9031a84ba\"},{\"content\":{\"connectorIds\":[\"Out1\",\"Out2\",\"Out3\",\"Out4\"],\"side\":\"RIGHT\"},\"type\":\"ConnectorPlacement.EquallySpacedRectSide\",\"uuid\":\"ca7acdc8-82b2-4681-aa13-89f67544921e\"},{\"content\":{\"connectorIds\":[],\"side\":\"TOP\"},\"type\":\"ConnectorPlacement.EquallySpacedRectSide\",\"uuid\":\"8b24d124-fa07-455d-a189-f258fbea822f\"}]},\"type\":\"ConnectorPlacement.EquallySpacedConnector\",\"uuid\":\"6802f4c9-cf5e-4fdc-ad1f-26d27f7bb24e\"}],\"packageUris\":[\"http://schema.mathworks.com/mf0/Connector/R2020b\"],\"version\":\"1.0\"}"
  pulse : Subsystem  ReferencedSubsystem=pulse
      settings: PortSchema="{\"entries\":[{\"content\":{\"sides\":[{\"content\":{\"connectorIds\":[\"In1\"]},\"type\":\"ConnectorPlacement.EquallySpacedRectSide\",\"uuid\":\"afba3d91-0482-4080-ad5b-85efc01ac040\"},{\"content\":{\"connectorIds\":[\"Out2\",\"Out1\"],\"side\":\"RIGHT\"},\"type\":\"ConnectorPlacement.EquallySpacedRectSide\",\"uuid\":\"57b935d0-c216-4bff-97b2-7e56f57779e2\"},{\"content\":{\"connectorIds\":[],\"side\":\"TOP\"},\"type\":\"ConnectorPlacement.EquallySpacedRectSide\",\"uuid\":\"5aece345-1746-4a20-9168-a2305e1b4a11\"}]},\"type\":\"ConnectorPlacement.EquallySpacedConnector\",\"uuid\":\"be92ca3f-dcfa-40d5-9481-c81581f266b6\"}],\"packageUris\":[\"http://schema.mathworks.com/mf0/Connector/R2020b\"],\"version\":\"1.0\"}"
  sclDeb : Subsystem  Commented=through  ReferencedSubsystem=debounce
  sco_slave_sel : Truth Table  TreatAsAtomicUnit=on
  sdaDeb : Subsystem  Commented=through  ReferencedSubsystem=debounce
  sdo_master_sel : Truth Table  TreatAsAtomicUnit=on
      settings: PortSchema="{\"entries\":[{\"content\":{\"sides\":[{\"content\":{\"connectorIds\":[\"In2\",\"In1\",\"In3\"]},\"type\":\"ConnectorPlacement.EquallySpacedRectSide\",\"uuid\":\"8adf670c-77d8-45e4-aece-f21f647edf41\"},{\"content\":{\"connectorIds\":[\"Out1\"],\"side\":\"RIGHT\"},\"type\":\"ConnectorPlacement.EquallySpacedRectSide\",\"uuid\":\"d41576bb-4bae-492b-8138-e8c2031f8f0a\"},{\"content\":{\"connectorIds\":[],\"side\":\"TOP\"},\"type\":\"ConnectorPlacement.EquallySpacedRectSide\",\"uuid\":\"0ee46126-e405-49c6-b738-dac8b4325e4e\"}]},\"type\":\"ConnectorPlacement.EquallySpacedConnector\",\"uuid\":\"ca60e9e9-b942-4103-97b2-e194946e788c\"}],\"packageUris\":[\"http://schema.mathworks.com/mf0/Connector/R2020b\"],\"version\":\"1.0\"}"
  sdo_slave_sel : Truth Table  TreatAsAtomicUnit=on
  sco_master : Outport
  sdo_master : Outport  Port=2
  sco_slave : Outport  Port=3
  sdo_slave : Outport  Port=4
  last_byte : Outport  Port=5
  wires:
  Constant1/1 -> i2c_slave_serializer/3
  sdaDeb/1 -> Data Type Conversion3/1, sdo_slave_sel/2(w), pulse/1
  Data Type Conversion2/1 -> i2c_slave_serializer/1
  Constant/1 -> i2c_slave_serializer/4
  sclDeb/1 -> Data Type Conversion2/1, sco_slave_sel/2(w), Stop/1, Start/2, NOT1/1
  Data Type Conversion3/1 -> i2c_slave_serializer/2
  pulse/1 -> Stop/2
  pulse/2 -> Start/1
  Start/1 -> Unit Delay Enabled Resettable Synchronous1/3
  i2c_slave_serializer/3 -> MuxSelReg/1
  Constant2/1 -> Unit Delay Enabled Resettable Synchronous1/1
  Unit Delay Enabled Resettable Synchronous1/1 -> AND3/1
  Stop/1 -> AND3/2
  Constant3/1 -> sco_master/1
  NOT/1 -> Unit Delay Enabled Resettable Synchronous1/2
  MuxSelReg/1 -> Delay/1
  sdi_slave/1 -> sdo_master_sel/2(v)
  i2c_slave_serializer/1 -> Data Type Conversion1/1, NOT/1
  sci_master/1 -> sclDeb/1
  sdi_master/1 -> sdaDeb/1
  sco_slave_sel/1(y) -> sco_slave/1
  sdo_slave_sel/1(y) -> sdo_slave/1
  NOT1/1 -> HDL Counter/1
  Compare To Constant/1 -> HDL Counter/2
  HDL Counter/1 -> Compare To Constant1/1
  Compare To Constant1/1 -> Unit Delay/1
  Unit Delay/1 -> MuxSelReg/3
  Unit Delay1/1 -> Compare To Constant/1
  Data Type Conversion1/1 -> sdo_master_sel/1(w), Unit Delay2/1
  AND/1 -> sdo_master/1
  sdo_master_sel/1(y) -> AND/2
  Unit Delay2/1 -> AND/1
  AND3/1 -> MuxSelReg/2
  Delay/1 -> sdo_master_sel/3(u), Unit Delay1/1, last_byte/1, sco_slave_sel/1(u), sdo_slave_sel/1(u)

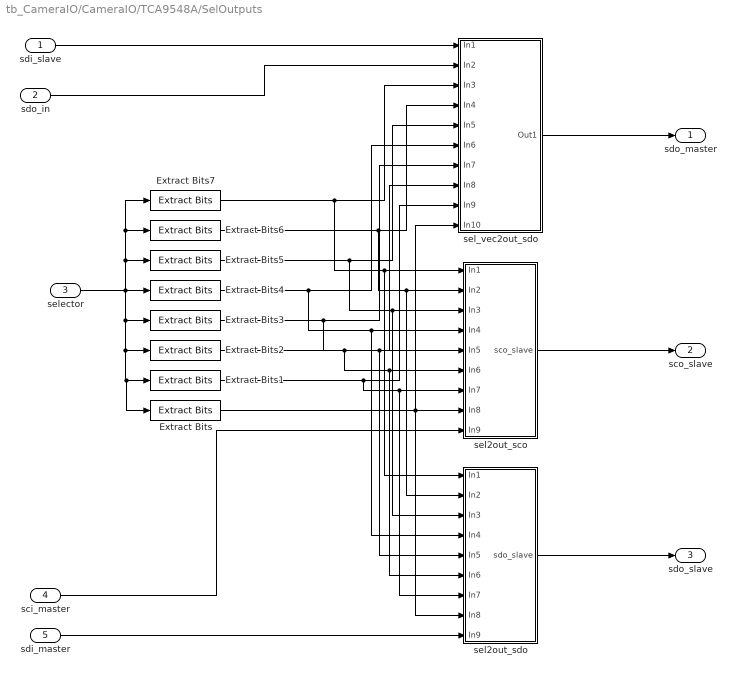
== system tb_CameraIO/CameraIO/TCA9548A/SelOutputs ==
  sdi_slave : Inport
  sdo_in : Inport  Port=2
  selector : Inport  Port=3
  sci_master : Inport  Port=4
  sdi_master : Inport  Port=5
  Extract Bits : simulink/Logic and Bit Operations/Extract Bits  bitsToExtract=Range of bits  numBits=8  bitIdxRange=7  outScalingMode=Treat bit field as an integer
  Extract Bits1 : simulink/Logic and Bit Operations/Extract Bits  bitsToExtract=Range of bits  numBits=8  bitIdxRange=6  outScalingMode=Treat bit field as an integer
  Extract Bits2 : simulink/Logic and Bit Operations/Extract Bits  bitsToExtract=Range of bits  numBits=8  bitIdxRange=5  outScalingMode=Treat bit field as an integer
  Extract Bits3 : simulink/Logic and Bit Operations/Extract Bits  bitsToExtract=Range of bits  numBits=8  bitIdxRange=4  outScalingMode=Treat bit field as an integer
  Extract Bits4 : simulink/Logic and Bit Operations/Extract Bits  bitsToExtract=Range of bits  numBits=8  bitIdxRange=3  outScalingMode=Treat bit field as an integer
  Extract Bits5 : simulink/Logic and Bit Operations/Extract Bits  bitsToExtract=Range of bits  numBits=8  bitIdxRange=2  outScalingMode=Treat bit field as an integer
  Extract Bits6 : simulink/Logic and Bit Operations/Extract Bits  bitsToExtract=Range of bits  numBits=8  bitIdxRange=1  outScalingMode=Treat bit field as an integer
  Extract Bits7 : simulink/Logic and Bit Operations/Extract Bits  bitsToExtract=Range of bits  numBits=8  bitIdxRange=0  outScalingMode=Treat bit field as an integer
  sel2out_sco : Subsystem
  sel2out_sdo : Subsystem
  sel_vec2out_sdo : Subsystem
  sdo_master : Outport
  sco_slave : Outport  Port=2
  sdo_slave : Outport  Port=3
  wires:
  Extract Bits1/1 -> sel_vec2out_sdo/9(In9), sel2out_sdo/7(In7), sel2out_sco/7(In7)
  selector/1 -> Extract Bits7/1, Extract Bits6/1, Extract Bits5/1, Extract Bits/1, Extract Bits1/1, Extract Bits2/1, Extract Bits3/1, Extract Bits4/1
  sdi_slave/1 -> sel_vec2out_sdo/1(In1)
  Extract Bits5/1 -> sel_vec2out_sdo/5(In5), sel2out_sdo/3(In3), sel2out_sco/3(In3)
  Extract Bits7/1 -> sel_vec2out_sdo/3(In3), sel2out_sco/1(In1), sel2out_sdo/1(In1)
  Extract Bits3/1 -> sel_vec2out_sdo/7(In7), sel2out_sco/5(In5), sel2out_sdo/5(In5)
  Extract Bits/1 -> sel2out_sdo/8(In8), sel2out_sco/8(In8), sel_vec2out_sdo/10(In10)
  Extract Bits2/1 -> sel_vec2out_sdo/8(In8), sel2out_sdo/6(In6), sel2out_sco/6(In6)
  Extract Bits6/1 -> sel_vec2out_sdo/4(In4), sel2out_sdo/2(In2), sel2out_sco/2(In2)
  Extract Bits4/1 -> sel_vec2out_sdo/6(In6), sel2out_sdo/4(In4), sel2out_sco/4(In4)
  sdo_in/1 -> sel_vec2out_sdo/2(In2)
  sdi_master/1 -> sel2out_sdo/9(In9)
  sel_vec2out_sdo/1(Out1) -> sdo_master/1
  sci_master/1 -> sel2out_sco/9(In9)
  sel2out_sco/1(sco_slave) -> sco_slave/1
  sel2out_sdo/1(sdo_slave) -> sdo_slave/1

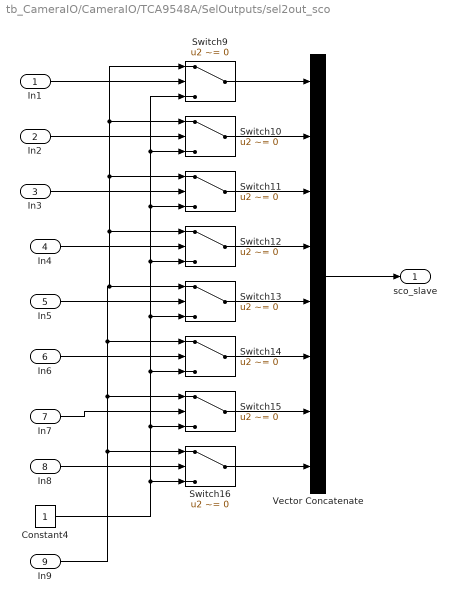
== system tb_CameraIO/CameraIO/TCA9548A/SelOutputs/sel2out_sco ==
  In1 : Inport
  In2 : Inport  Port=2
  In3 : Inport  Port=3
  In4 : Inport  Port=4
  In5 : Inport  Port=5
  In6 : Inport  Port=6
  In7 : Inport  Port=7
  In8 : Inport  Port=8
  In9 : Inport  Port=9
  Constant4 : Constant  OutDataTypeStr=boolean  SampleTime=-1
  Switch{9..16} (8 alike) : Switch  Criteria=u2 ~= 0  SaturateOnIntegerOverflow=off  InputSameDT=off
  Vector Concatenate : Concatenate  NumInputs=8
  sco_slave : Outport
  wires:
  Switch9/1 -> Vector Concatenate/1
  Vector Concatenate/1 -> sco_slave/1
  Constant4/1 -> Switch14/3, Switch9/3, Switch10/3, Switch11/3, Switch12/3, Switch13/3, Switch15/3, Switch16/3
  In6/1 -> Switch14/2
  In9/1 -> Switch9/1, Switch10/1, Switch11/1, Switch12/1, Switch13/1, Switch14/1, Switch15/1, Switch16/1
  Switch11/1 -> Vector Concatenate/3
  Switch13/1 -> Vector Concatenate/5
  In3/1 -> Switch11/2
  In5/1 -> Switch13/2
  In7/1 -> Switch15/2
  Switch16/1 -> Vector Concatenate/8
  Switch14/1 -> Vector Concatenate/6
  Switch10/1 -> Vector Concatenate/2
  Switch12/1 -> Vector Concatenate/4
  Switch15/1 -> Vector Concatenate/7
  In2/1 -> Switch10/2
  In1/1 -> Switch9/2
  In8/1 -> Switch16/2
  In4/1 -> Switch12/2

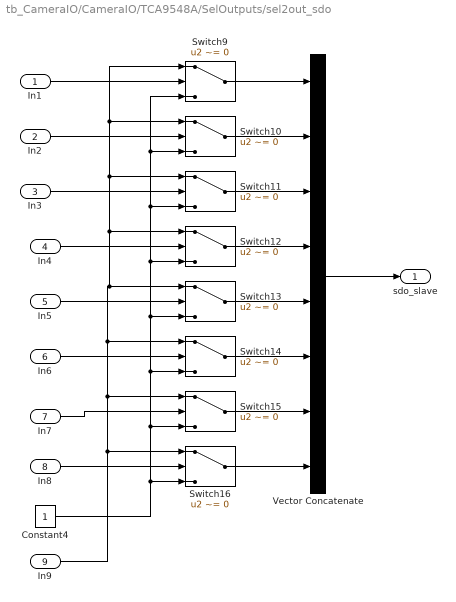
== system tb_CameraIO/CameraIO/TCA9548A/SelOutputs/sel2out_sdo ==
  In1 : Inport
  In2 : Inport  Port=2
  In3 : Inport  Port=3
  In4 : Inport  Port=4
  In5 : Inport  Port=5
  In6 : Inport  Port=6
  In7 : Inport  Port=7
  In8 : Inport  Port=8
  In9 : Inport  Port=9
  Constant4 : Constant  OutDataTypeStr=boolean  SampleTime=-1
  Switch{9..16} (8 alike) : Switch  Criteria=u2 ~= 0  SaturateOnIntegerOverflow=off  InputSameDT=off
  Vector Concatenate : Concatenate  NumInputs=8
  sdo_slave : Outport
  wires:
  Switch9/1 -> Vector Concatenate/1
  Vector Concatenate/1 -> sdo_slave/1
  Constant4/1 -> Switch14/3, Switch9/3, Switch10/3, Switch11/3, Switch12/3, Switch13/3, Switch15/3, Switch16/3
  In6/1 -> Switch14/2
  In9/1 -> Switch9/1, Switch10/1, Switch11/1, Switch12/1, Switch13/1, Switch14/1, Switch15/1, Switch16/1
  Switch11/1 -> Vector Concatenate/3
  Switch13/1 -> Vector Concatenate/5
  In3/1 -> Switch11/2
  In5/1 -> Switch13/2
  In7/1 -> Switch15/2
  Switch16/1 -> Vector Concatenate/8
  Switch14/1 -> Vector Concatenate/6
  Switch10/1 -> Vector Concatenate/2
  Switch12/1 -> Vector Concatenate/4
  Switch15/1 -> Vector Concatenate/7
  In2/1 -> Switch10/2
  In1/1 -> Switch9/2
  In8/1 -> Switch16/2
  In4/1 -> Switch12/2

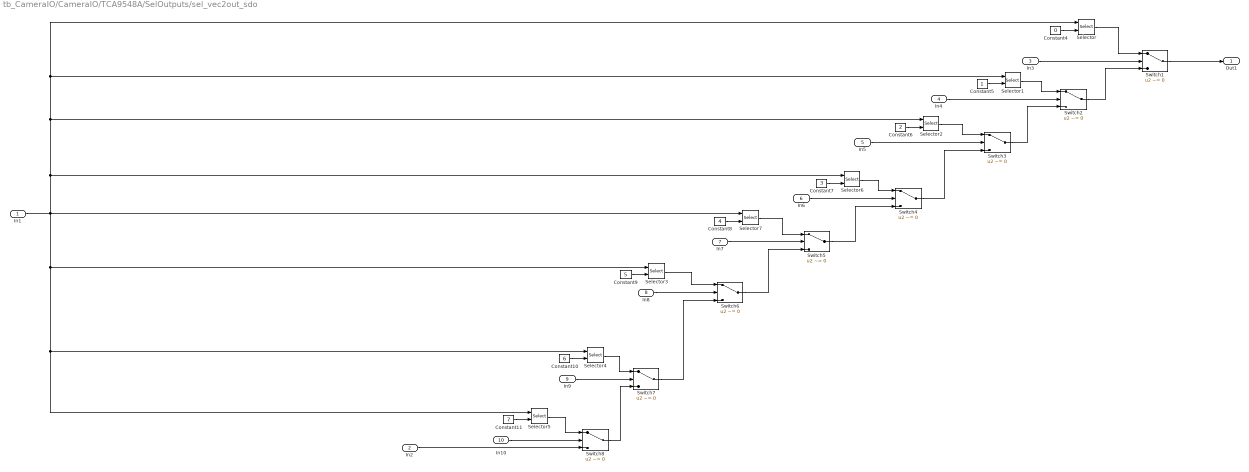
== system tb_CameraIO/CameraIO/TCA9548A/SelOutputs/sel_vec2out_sdo ==
  In1 : Inport
  In2 : Inport  Port=2
  In3 : Inport  Port=3
  In4 : Inport  Port=4
  In5 : Inport  Port=5
  In6 : Inport  Port=6
  In7 : Inport  Port=7
  In8 : Inport  Port=8
  In9 : Inport  Port=9
  In10 : Inport  Port=10
  Constant10 : Constant  Value=6  OutDataTypeStr=uint8  SampleTime=-1
  Constant11 : Constant  Value=7  OutDataTypeStr=uint8  SampleTime=-1
  Constant4 : Constant  Value=0  OutDataTypeStr=uint8  SampleTime=-1
  Constant5 : Constant  OutDataTypeStr=uint8  SampleTime=-1
  Constant6 : Constant  Value=2  OutDataTypeStr=uint8  SampleTime=-1
  Constant7 : Constant  Value=3  OutDataTypeStr=uint8  SampleTime=-1
  Constant8 : Constant  Value=4  OutDataTypeStr=uint8  SampleTime=-1
  Constant9 : Constant  Value=5  OutDataTypeStr=uint8  SampleTime=-1
  Selector{,1..7} (8 alike) : Selector  IndexMode=Zero-based  IndexOptions=Index vector (port)  Indices=0  OutputSizes=1
  Switch{1..8} (8 alike) : Switch  Criteria=u2 ~= 0  SaturateOnIntegerOverflow=off  InputSameDT=off
  Out1 : Outport
  wires:
  Selector4/1 -> Switch7/1
  In10/1 -> Switch8/2
  Switch7/1 -> Switch6/3
  Switch5/1 -> Switch4/3
  Selector3/1 -> Switch6/1
  Selector5/1 -> Switch8/1
  In7/1 -> Switch5/2
  In3/1 -> Switch1/2
  Selector1/1 -> Switch2/1
  In6/1 -> Switch4/2
  Selector2/1 -> Switch3/1
  In8/1 -> Switch6/2
  Switch2/1 -> Switch1/3
  Switch3/1 -> Switch2/3
  Switch1/1 -> Out1/1
  Switch4/1 -> Switch3/3
  Switch8/1 -> Switch7/3
  Selector6/1 -> Switch4/1
  In2/1 -> Switch8/3
  Switch6/1 -> Switch5/3
  Selector/1 -> Switch1/1
  In9/1 -> Switch7/2
  Selector7/1 -> Switch5/1
  In4/1 -> Switch2/2
  In5/1 -> Switch3/2
  Constant6/1 -> Selector2/2
  Constant7/1 -> Selector6/2
  Constant8/1 -> Selector7/2
  Constant4/1 -> Selector/2
  Constant9/1 -> Selector3/2
  Constant5/1 -> Selector1/2
  Constant11/1 -> Selector5/2
  Constant10/1 -> Selector4/2
  In1/1 -> Selector7/1, Selector/1, Selector1/1, Selector2/1, Selector6/1, Selector4/1, Selector5/1, Selector3/1

== matlab function tb_CameraIO/CameraIO/TCA9548A/sco_slave_sel ==
  data: u input; y output; w input
function y = fcn(u, w)

aVarTruthTableCondition_1 = false;
aVarTruthTableCondition_2 = false;
aVarTruthTableCondition_3 = false;
aVarTruthTableCondition_4 = false;
aVarTruthTableCondition_5 = false;
aVarTruthTableCondition_6 = false;
aVarTruthTableCondition_7 = false;
aVarTruthTableCondition_8 = false;


% sel 1

aVarTruthTableCondition_1 = logical(bitget(u,1));

% sel 2

aVarTruthTableCondition_2 = logical(bitget(u,2));

% sel 3

aVarTruthTableCondition_3 = logical(bitget(u,3));

% sel 4

aVarTruthTableCondition_4 = logical(bitget(u,4));

% sel 5

aVarTruthTableCondition_5 = logical(bitget(u,5));

% sel 6

aVarTruthTableCondition_6 = logical(bitget(u,6));

% sel 7

aVarTruthTableCondition_7 = logical(bitget(u,7));

% sel 8

aVarTruthTableCondition_8 = logical(bitget(u,8));

if (aVarTruthTableCondition_1)
    aFcnTruthTableAction_1();
elseif (aVarTruthTableCondition_2)
    aFcnTruthTableAction_2();
elseif (aVarTruthTableCondition_3)
    aFcnTruthTableAction_3();
elseif (aVarTruthTableCondition_4)
    aFcnTruthTableAction_4();
elseif (aVarTruthTableCondition_5)
    aFcnTruthTableAction_5();
elseif (aVarTruthTableCondition_6)
    aFcnTruthTableAction_6();
elseif (aVarTruthTableCondition_7)
    aFcnTruthTableAction_7();
elseif (aVarTruthTableCondition_8)
    aFcnTruthTableAction_8();
else % Default
    aFcnTruthTableAction_9();
end

function aFcnTruthTableAction_1()

% sel 1

y = boolean(ones(8,1));
y(1) = w;

function aFcnTruthTableAction_2()

% sel 2

y = boolean(ones(8,1));
y(2) = w;

function aFcnTruthTableAction_3()

% sel 3

y = boolean(ones(8,1));
y(3) = w;

function aFcnTruthTableAction_4()

% sel 4

y = boolean(ones(8,1));
y(4) = w;

function aFcnTruthTableAction_5()

% sel 5

y = boolean(ones(8,1));
y(5) = w;

function aFcnTruthTableAction_6()

% sel 6

y = boolean(ones(8,1));
y(6) = w;

function aFcnTruthTableAction_7()

% sel 7

y = boolean(ones(8,1));
y(7) = w;

function aFcnTruthTableAction_8()

% sel 8

y = boolean(ones(8,1));
y(8) = w;

function aFcnTruthTableAction_9()

% sel none

y = boolean(ones(8,1));

== matlab function tb_CameraIO/CameraIO/TCA9548A/sdo_master_sel ==
  data: w input; v input; u input; y output
function y = fcn(w, v, u)

aVarTruthTableCondition_1 = false;
aVarTruthTableCondition_2 = false;
aVarTruthTableCondition_3 = false;
aVarTruthTableCondition_4 = false;
aVarTruthTableCondition_5 = false;
aVarTruthTableCondition_6 = false;
aVarTruthTableCondition_7 = false;
aVarTruthTableCondition_8 = false;


% sel 1

aVarTruthTableCondition_1 = logical(bitget(u,1));

% sel 2

aVarTruthTableCondition_2 = logical(bitget(u,2));

% sel 3

aVarTruthTableCondition_3 = logical(bitget(u,3));

% sel 4

aVarTruthTableCondition_4 = logical(bitget(u,4));

% sel 5

aVarTruthTableCondition_5 = logical(bitget(u,5));

% sel 6

aVarTruthTableCondition_6 = logical(bitget(u,6));

% sel 7

aVarTruthTableCondition_7 = logical(bitget(u,7));

% sel 8

aVarTruthTableCondition_8 = logical(bitget(u,8));

if (aVarTruthTableCondition_1)
    aFcnTruthTableAction_1();
elseif (aVarTruthTableCondition_2)
    aFcnTruthTableAction_2();
elseif (aVarTruthTableCondition_3)
    aFcnTruthTableAction_3();
elseif (aVarTruthTableCondition_4)
    aFcnTruthTableAction_4();
elseif (aVarTruthTableCondition_5)
    aFcnTruthTableAction_5();
elseif (aVarTruthTableCondition_6)
    aFcnTruthTableAction_6();
elseif (aVarTruthTableCondition_7)
    aFcnTruthTableAction_7();
elseif (aVarTruthTableCondition_8)
    aFcnTruthTableAction_8();
else % Default
    aFcnTruthTableAction_9();
end

function aFcnTruthTableAction_1()

% sel 1

y = v(1);

function aFcnTruthTableAction_2()

% sel 2

y = v(2);

function aFcnTruthTableAction_3()

% sel 3

y = v(3);

function aFcnTruthTableAction_4()

% sel 4

y = v(4);

function aFcnTruthTableAction_5()

% sel 5

y = v(5);

function aFcnTruthTableAction_6()

% sel 6

y = v(6);

function aFcnTruthTableAction_7()

% sel 7

y = v(7);

function aFcnTruthTableAction_8()

% sel 8

y = v(8);

function aFcnTruthTableAction_9()

% sel none

y = true;

== matlab function tb_CameraIO/CameraIO/TCA9548A/sdo_slave_sel ==
  data: u input; y output; w input
function y = fcn(u, w)

aVarTruthTableCondition_1 = false;
aVarTruthTableCondition_2 = false;
aVarTruthTableCondition_3 = false;
aVarTruthTableCondition_4 = false;
aVarTruthTableCondition_5 = false;
aVarTruthTableCondition_6 = false;
aVarTruthTableCondition_7 = false;
aVarTruthTableCondition_8 = false;


% sel 1

aVarTruthTableCondition_1 = logical(bitget(u,1));

% sel 2

aVarTruthTableCondition_2 = logical(bitget(u,2));

% sel 3

aVarTruthTableCondition_3 = logical(bitget(u,3));

% sel 4

aVarTruthTableCondition_4 = logical(bitget(u,4));

% sel 5

aVarTruthTableCondition_5 = logical(bitget(u,5));

% sel 6

aVarTruthTableCondition_6 = logical(bitget(u,6));

% sel 7

aVarTruthTableCondition_7 = logical(bitget(u,7));

% sel 8

aVarTruthTableCondition_8 = logical(bitget(u,8));

if (aVarTruthTableCondition_1)
    aFcnTruthTableAction_1();
elseif (aVarTruthTableCondition_2)
    aFcnTruthTableAction_2();
elseif (aVarTruthTableCondition_3)
    aFcnTruthTableAction_3();
elseif (aVarTruthTableCondition_4)
    aFcnTruthTableAction_4();
elseif (aVarTruthTableCondition_5)
    aFcnTruthTableAction_5();
elseif (aVarTruthTableCondition_6)
    aFcnTruthTableAction_6();
elseif (aVarTruthTableCondition_7)
    aFcnTruthTableAction_7();
elseif (aVarTruthTableCondition_8)
    aFcnTruthTableAction_8();
else % Default
    aFcnTruthTableAction_9();
end

function aFcnTruthTableAction_1()

% sel 1

y = boolean(ones(8,1));
y(1) = w;

function aFcnTruthTableAction_2()

% sel 2

y = boolean(ones(8,1));
y(2) = w;

function aFcnTruthTableAction_3()

% sel 3

y = boolean(ones(8,1));
y(3) = w;

function aFcnTruthTableAction_4()

% sel 4

y = boolean(ones(8,1));
y(4) = w;

function aFcnTruthTableAction_5()

% sel 5

y = boolean(ones(8,1));
y(5) = w;

function aFcnTruthTableAction_6()

% sel 6

y = boolean(ones(8,1));
y(6) = w;

function aFcnTruthTableAction_7()

% sel 7

y = boolean(ones(8,1));
y(7) = w;

function aFcnTruthTableAction_8()

% sel 8

y = boolean(ones(8,1));
y(8) = w;

function aFcnTruthTableAction_9()

% sel none

y = boolean(ones(8,1));
